simulink model "EPD629_WilliamsJ_AS06_Simulink"  (R2021b)
settings: Solver=VariableStepAuto  StartTime=0.0  StopTime=10.0  MaxStep=0.01  RelTol=1e-3
values from neighbouring files (symbols this model uses):
  AirGasConstant_kJpkgK = 0.287    [EPD629_WilliamsJ_AS06.m]
  AirToFuelEquivalenceRatio_frac = 1    [EPD629_WilliamsJ_AS06.m]
  AmbientPressure_kPa = 98    [EPD629_WilliamsJ_AS06.m]
  CrankAngleIVCToTDC_deg = 170    [EPD629_WilliamsJ_AS06.m]
  DischargeCoefficient_frac = 0.7    [EPD629_WilliamsJ_AS06.m]
  EngineDisplacement_L = 2.77    [EPD629_WilliamsJ_AS06.m]
  EngineInertia_kgm2 = 0.2    [EPD629_WilliamsJ_AS06.m]
  EngineMotoringFrictionData_Nm = Beta_0 + Beta_2*Omega_e.^2    [EPD629_WilliamsJ_AS06.m]
  EngineSpeedBreakpoints_rpm = 400:200:5000    [EPD629_WilliamsJ_AS06.m]
  FuelLowerHeatingValue_kJpkg = 44000    [EPD629_WilliamsJ_AS06.m]
  InletAirTemperature_K = 298    [EPD629_WilliamsJ_AS06.m]
  IntakeManifoldVolume_L = 5.8    [EPD629_WilliamsJ_AS06.m]
  ManifoldAirTemperature_K = 340    [EPD629_WilliamsJ_AS06.m]
  ManifoldPressureBreakpoints_kPa = 5:5:100    [EPD629_WilliamsJ_AS06.m]
  StoichiometricAFR_frac = 14.7    [EPD629_WilliamsJ_AS06.m]
  ThermodynamicEfficiencyData_frac = Eta_0 + Eta_1*Omega_e + Eta_2*Omega_e.^2    [EPD629_WilliamsJ_AS06.m]
  ThrottleAreaBreakpoints_pct = ThrottleAreaData_pct    [EPD629_WilliamsJ_AS06.m]
  ThrottleAreaData_pct = 100 * ThrottleArea_mm2 / WideOpenThrottleArea_mm2    [EPD629_WilliamsJ_AS06.m]
  ThrottleFlowFunctionData_frac = PR.^(1/RatioOfSpecificHeats_frac) .*      sqrt( 2 * RatioOfSpecificHeats_frac / (RatioOfSpecificHeats_frac - 1) .*      (1 - PR.^((RatioOfSpecificHeats_frac - 1) / RatioOfSpecificHeats_frac)) )    [EPD629_WilliamsJ_AS06.m]
  ThrottlePositionBreakpoints_pct = 0:100    [EPD629_WilliamsJ_AS06.m]
  ThrottlePositionData_pct = ThrottlePositionBreakpoints_pct    [EPD629_WilliamsJ_AS06.m]
  ThrottlePressureRatioBreakpoints_frac = 0:0.01:1    [EPD629_WilliamsJ_AS06.m]
  WideOpenThrottleArea_mm2 = ThrottleArea_mm2(end)    [EPD629_WilliamsJ_AS06.m]
undefined symbols (not defined in the file or in its folder): VolumetricEfficiencyData_frac
settings Model: Creator=Justin  LastModifiedBy=Justin

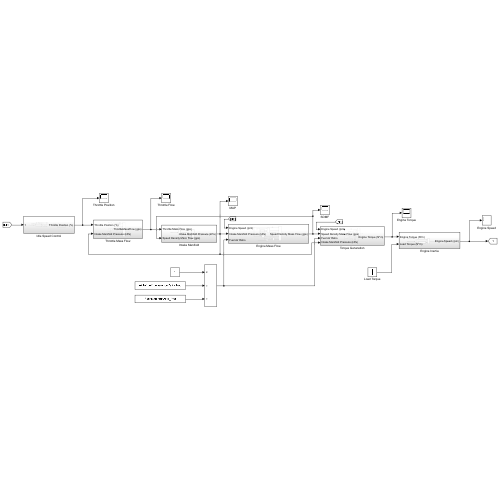
[thumbnail: Simulink's stored preview of the top-level diagram]
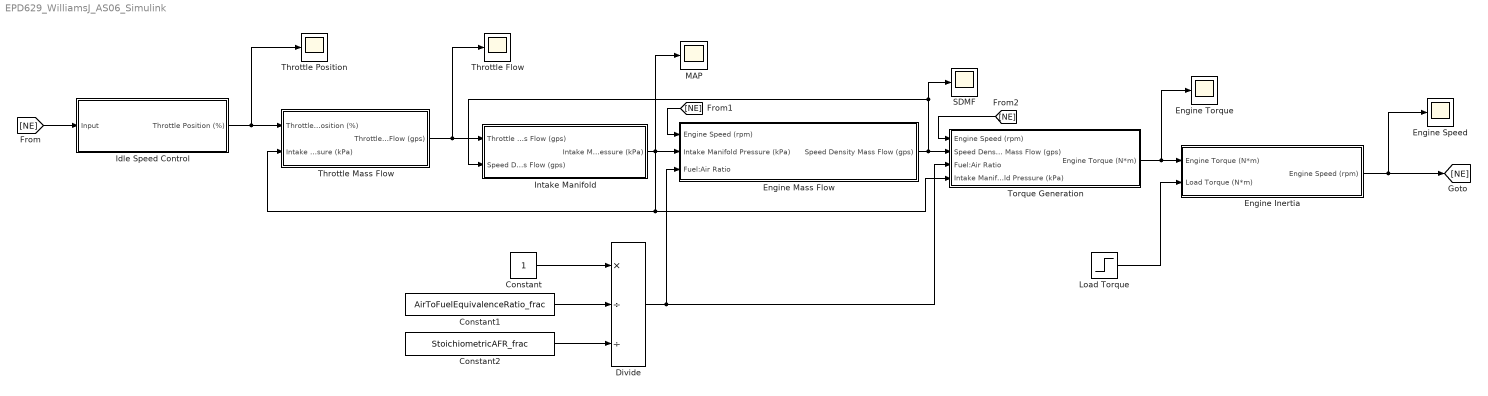
== system EPD629_WilliamsJ_AS06_Simulink ==
  Constant : Constant
  Constant1 : Constant  Value=AirToFuelEquivalenceRatio_frac
  Constant2 : Constant  Value=StoichiometricAFR_frac
  Divide : Product  Inputs=*//
  Engine Inertia : Subsystem
  Engine Mass Flow : Subsystem
  Engine Speed : Scope
  Engine Torque : Scope
  Idle Speed Control : Subsystem
  Intake Manifold : Subsystem
  Load Torque : Step  Time=5  Before=15  After=25  SampleTime=0
  MAP : Scope
  SDMF : Scope
  Throttle Flow : Scope
  Throttle Mass Flow : Subsystem
  Throttle Position : Scope
  Torque Generation : Subsystem
  wires:
  Constant/1 -> Divide/1
  Constant1/1 -> Divide/2
  Constant2/1 -> Divide/3
  Divide/1 -> Engine Mass Flow/3(Fuel:Air Ratio), Torque Generation/3(Fuel:Air Ratio)
  Load Torque/1 -> Engine Inertia/2(Load Torque (N*m))
  Idle Speed Control/1(Throttle Position (%)) -> Throttle Position/1, Throttle Mass Flow/1(Throttle Position (%))
  Throttle Mass Flow/1(ThrottleMassFlow (gps)) -> Throttle Flow/1, Intake Manifold/1(Throttle Mass Flow (gps))
  Intake Manifold/1(Intake Manifold Pressure (kPa)) -> Torque Generation/4(Intake Manifold Pressure (kPa)), Throttle Mass Flow/2(Intake Manifold Pressure (kPa)), MAP/1, Engine Mass Flow/2(Intake Manifold Pressure (kPa))
  Engine Mass Flow/1(Speed Density Mass Flow (gps)) -> SDMF/1, Intake Manifold/2(Speed Density Mass Flow (gps)), Torque Generation/2(Speed Density Mass Flow (gps))
  Torque Generation/1(Engine Torque (N*m)) -> Engine Torque/1, Engine Inertia/1(Engine Torque (N*m))
  Engine Inertia/1(Engine Speed (rpm)) -> [NE], Engine Speed/1
  [NE] -> Idle Speed Control/1(Input)
  [NE] -> Engine Mass Flow/1(Engine Speed (rpm))
  [NE] -> Torque Generation/1(Engine Speed (rpm))

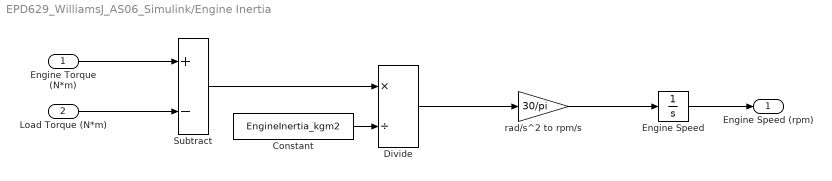
== system EPD629_WilliamsJ_AS06_Simulink/Engine Inertia ==
  Engine Torque (N*m) : Inport
  Load Torque (N*m) : Inport  Port=2
  Constant : Constant  Value=EngineInertia_kgm2
  Divide : Product  Inputs=*/
  Engine Speed : Integrator  InitialCondition=600  LimitOutput=on  UpperSaturationLimit=5000  LowerSaturationLimit=0
  Subtract : Sum  Inputs=+-
  rad/s^2 to rpm/s : Gain  Gain=30/pi
  Engine Speed (rpm) : Outport
  wires:
  Engine Torque (N*m)/1 -> Subtract/1
  Load Torque (N*m)/1 -> Subtract/2
  Subtract/1 -> Divide/1
  Constant/1 -> Divide/2
  Divide/1 -> rad/s^2 to rpm/s/1
  rad/s^2 to rpm/s/1 -> Engine Speed/1
  Engine Speed/1 -> Engine Speed (rpm)/1

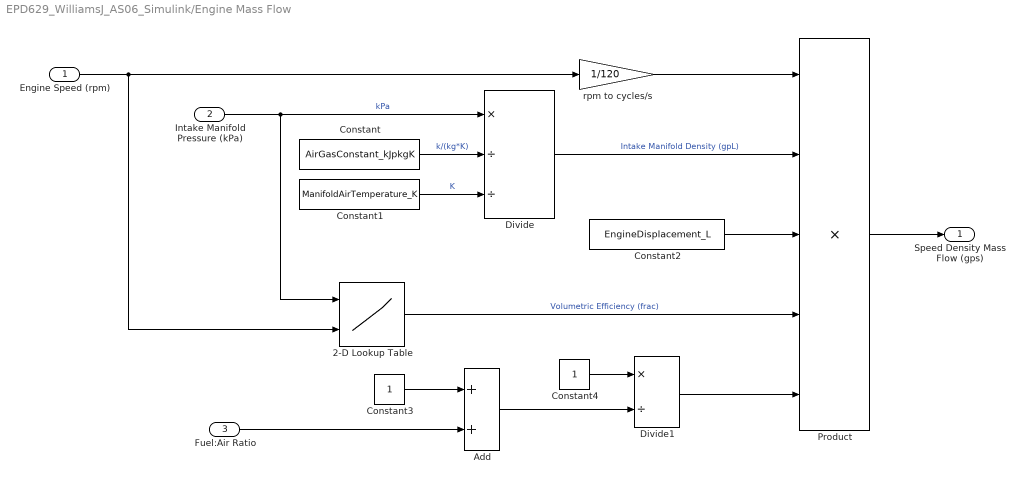
== system EPD629_WilliamsJ_AS06_Simulink/Engine Mass Flow ==
  Engine Speed (rpm) : Inport
  Intake Manifold Pressure (kPa) : Inport  Port=2
  Fuel:Air Ratio : Inport  Port=3
  2-D Lookup Table : Lookup_n-D  BreakpointsForDimension1=ManifoldPressureBreakpoints_kPa  BreakpointsForDimension2=EngineSpeedBreakpoints_rpm  Table=VolumetricEfficiencyData_frac  ExtrapMethod=Clip  UseLastTableValue=on  InternalRulePriority=Speed  RndMeth=Simplest  InputSameDT=on
      settings: InputPortMap=u0,u1
  Add : Sum
  Constant : Constant  Value=AirGasConstant_kJpkgK
  Constant1 : Constant  Value=ManifoldAirTemperature_K
  Constant2 : Constant  Value=EngineDisplacement_L
  Constant3 : Constant
  Constant4 : Constant
  Divide : Product  Inputs=*//
  Divide1 : Product  Inputs=*/
  Product : Product  Inputs=5
  rpm to cycles/s : Gain  Gain=1/120
  Speed Density Mass Flow (gps) : Outport
  wires:
  Engine Speed (rpm)/1 -> rpm to cycles/s/1, 2-D Lookup Table/2
  Intake Manifold Pressure (kPa)/1 -> Divide/1, 2-D Lookup Table/1  "kPa"
  Constant/1 -> Divide/2  "k/(kg*K)"
  Constant1/1 -> Divide/3  "K"
  rpm to cycles/s/1 -> Product/1
  Divide/1 -> Product/2  "Intake Manifold Density (gpL)"
  Constant2/1 -> Product/3
  2-D Lookup Table/1 -> Product/4  "Volumetric Efficiency (frac)"
  Constant3/1 -> Add/1
  Fuel:Air Ratio/1 -> Add/2
  Constant4/1 -> Divide1/1
  Add/1 -> Divide1/2
  Divide1/1 -> Product/5
  Product/1 -> Speed Density Mass Flow (gps)/1

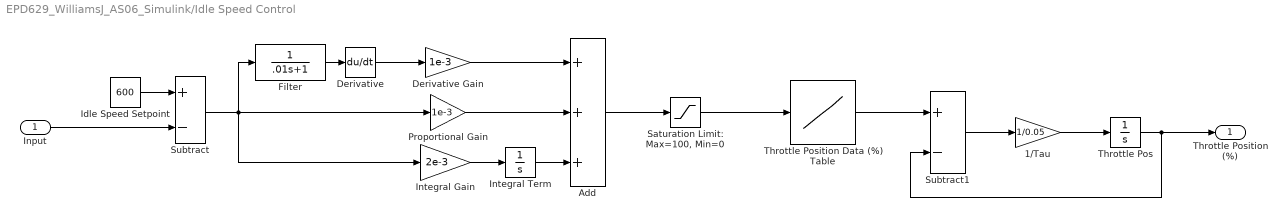
== system EPD629_WilliamsJ_AS06_Simulink/Idle Speed Control ==
  Input : Inport
  1/Tau : Gain  Gain=1/0.05
  Add : Sum  Inputs=+++
  Derivative : Derivative
  Derivative Gain : Gain  Gain=1e-3
  Filter : TransferFcn  Denominator=[.01 1]
  Idle Speed Setpoint : Constant  Value=600
  Integral Gain : Gain  Gain=2e-3
  Integral Term : Integrator  InitialCondition=0.6  LimitOutput=on  UpperSaturationLimit=100  LowerSaturationLimit=0
  Proportional Gain : Gain  Gain=1e-3
  "Saturation Limit: Max=100, Min=0" : Saturate  UpperLimit=100  LowerLimit=0
  Subtract : Sum  Inputs=+-
  Subtract1 : Sum  Inputs=+-
  Throttle Pos : Integrator  InitialCondition=1.7  LimitOutput=on  UpperSaturationLimit=100  LowerSaturationLimit=0
  Throttle Position Data (%) Table : Lookup_n-D  NumberOfTableDimensions=1  BreakpointsForDimension1=ThrottleAreaBreakpoints_pct  Table=ThrottlePositionData_pct  ExtrapMethod=Clip  UseLastTableValue=on  InternalRulePriority=Speed  RndMeth=Simplest  InputSameDT=on
  Throttle Position (%) : Outport
  wires:
  Idle Speed Setpoint/1 -> Subtract/1
  Filter/1 -> Derivative/1
  Subtract/1 -> Integral Gain/1, Filter/1, Proportional Gain/1
  Derivative/1 -> Derivative Gain/1
  Derivative Gain/1 -> Add/1
  Proportional Gain/1 -> Add/2
  Integral Gain/1 -> Integral Term/1
  Integral Term/1 -> Add/3
  Input/1 -> Subtract/2
  Add/1 -> "Saturation Limit: Max=100, Min=0"/1
  "Saturation Limit: Max=100, Min=0"/1 -> Throttle Position Data (%) Table/1
  Throttle Position Data (%) Table/1 -> Subtract1/1
  Subtract1/1 -> 1/Tau/1
  1/Tau/1 -> Throttle Pos/1
  Throttle Pos/1 -> Subtract1/2, Throttle Position (%)/1

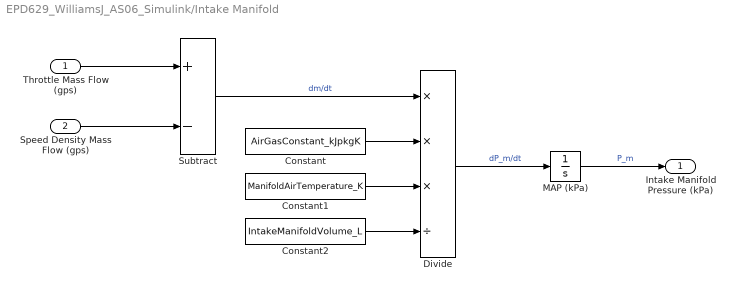
== system EPD629_WilliamsJ_AS06_Simulink/Intake Manifold ==
  Throttle Mass Flow (gps) : Inport
  Speed Density Mass Flow (gps) : Inport  Port=2
  Constant : Constant  Value=AirGasConstant_kJpkgK
  Constant1 : Constant  Value=ManifoldAirTemperature_K
  Constant2 : Constant  Value=IntakeManifoldVolume_L
  Divide : Product  Inputs=***/
  MAP (kPa) : Integrator  InitialCondition=33.5  LimitOutput=on  UpperSaturationLimit=110  LowerSaturationLimit=10
  Subtract : Sum  Inputs=+-
  Intake Manifold Pressure (kPa) : Outport
  wires:
  Throttle Mass Flow (gps)/1 -> Subtract/1
  Speed Density Mass Flow (gps)/1 -> Subtract/2
  Subtract/1 -> Divide/1  "dm/dt"
  Constant/1 -> Divide/2
  Constant1/1 -> Divide/3
  Constant2/1 -> Divide/4
  Divide/1 -> MAP (kPa)/1  "dP_m/dt"
  MAP (kPa)/1 -> Intake Manifold Pressure (kPa)/1  "P_m"

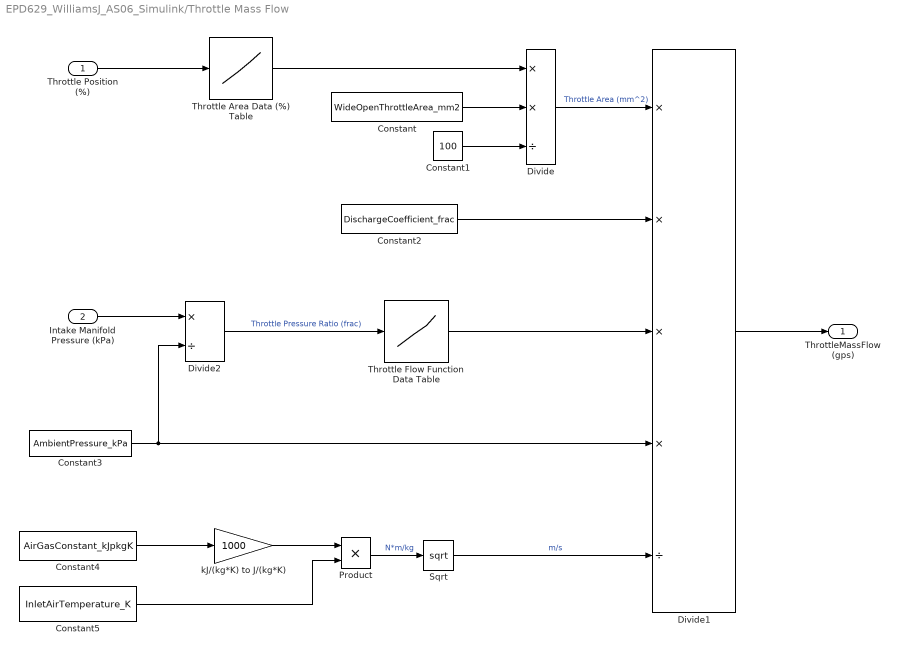
== system EPD629_WilliamsJ_AS06_Simulink/Throttle Mass Flow ==
  Throttle Position (%) : Inport
  Intake Manifold Pressure (kPa) : Inport  Port=2
  Constant : Constant  Value=WideOpenThrottleArea_mm2
  Constant1 : Constant  Value=100
  Constant2 : Constant  Value=DischargeCoefficient_frac
  Constant3 : Constant  Value=AmbientPressure_kPa
  Constant4 : Constant  Value=AirGasConstant_kJpkgK
  Constant5 : Constant  Value=InletAirTemperature_K
  Divide : Product  Inputs=**/
  Divide1 : Product  Inputs=****/
  Divide2 : Product  Inputs=*/
  Product : Product
  Sqrt : Sqrt  SaturateOnIntegerOverflow=on
  Throttle Area Data (%) Table : Lookup_n-D  NumberOfTableDimensions=1  BreakpointsForDimension1=ThrottlePositionBreakpoints_pct  Table=ThrottleAreaData_pct  ExtrapMethod=Clip  UseLastTableValue=on  InternalRulePriority=Speed  RndMeth=Simplest  InputSameDT=on
  Throttle Flow Function Data Table : Lookup_n-D  NumberOfTableDimensions=1  BreakpointsForDimension1=ThrottlePressureRatioBreakpoints_frac  Table=ThrottleFlowFunctionData_frac  ExtrapMethod=Clip  UseLastTableValue=on  InternalRulePriority=Speed  RndMeth=Simplest  InputSameDT=on
  kJ/(kg*K) to J/(kg*K) : Gain  Gain=1000
  ThrottleMassFlow (gps) : Outport
  wires:
  Throttle Position (%)/1 -> Throttle Area Data (%) Table/1
  Throttle Area Data (%) Table/1 -> Divide/1
  Constant/1 -> Divide/2
  Constant1/1 -> Divide/3
  Divide/1 -> Divide1/1  "Throttle Area (mm^2)"
  Constant2/1 -> Divide1/2
  Intake Manifold Pressure (kPa)/1 -> Divide2/1
  Constant3/1 -> Divide2/2, Divide1/4
  Throttle Flow Function Data Table/1 -> Divide1/3
  Divide2/1 -> Throttle Flow Function Data Table/1  "Throttle Pressure Ratio (frac)"
  Constant4/1 -> kJ/(kg*K) to J/(kg*K)/1
  kJ/(kg*K) to J/(kg*K)/1 -> Product/1
  Constant5/1 -> Product/2
  Product/1 -> Sqrt/1  "N*m/kg"
  Sqrt/1 -> Divide1/5  "m/s"
  Divide1/1 -> ThrottleMassFlow (gps)/1

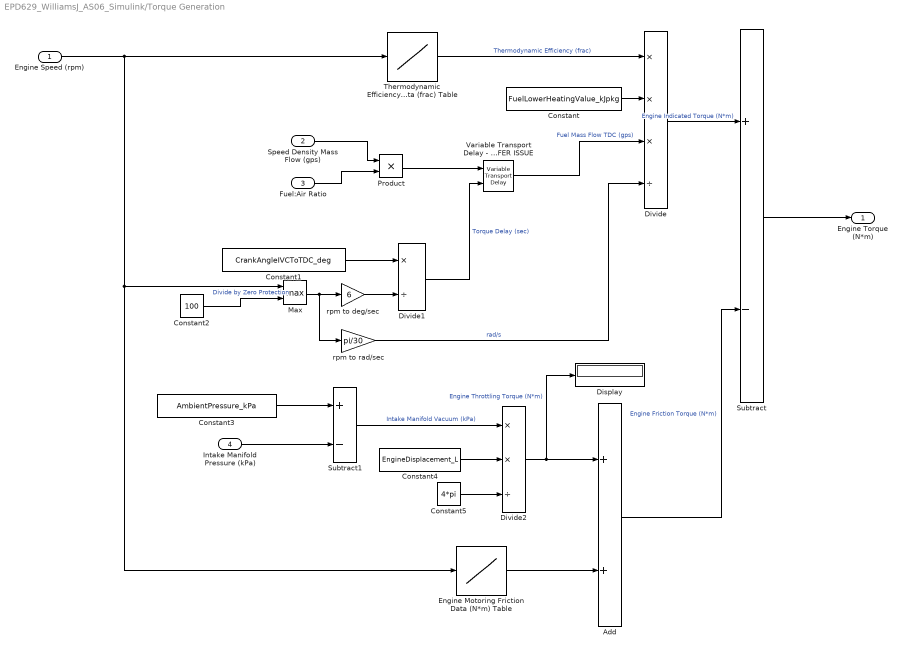
== system EPD629_WilliamsJ_AS06_Simulink/Torque Generation ==
  Engine Speed (rpm) : Inport
  Speed Density Mass Flow (gps) : Inport  Port=2
  Fuel:Air Ratio : Inport  Port=3
  Intake Manifold Pressure (kPa) : Inport  Port=4
  Add : Sum
  Constant : Constant  Value=FuelLowerHeatingValue_kJpkg
  Constant1 : Constant  Value=CrankAngleIVCToTDC_deg
  Constant2 : Constant  Value=100
  Constant3 : Constant  Value=AmbientPressure_kPa
  Constant4 : Constant  Value=EngineDisplacement_L
  Constant5 : Constant  Value=4*pi
  Display : Display
  Divide : Product  Inputs=***/
  Divide1 : Product  Inputs=*/
  Divide2 : Product  Inputs=**/
  Engine Motoring Friction Data (N*m) Table : Lookup_n-D  NumberOfTableDimensions=1  BreakpointsForDimension1=EngineSpeedBreakpoints_rpm  Table=EngineMotoringFrictionData_Nm  ExtrapMethod=Clip  UseLastTableValue=on  InternalRulePriority=Speed  RndMeth=Simplest  InputSameDT=on
  Max : MinMax  Function=max  Inputs=2
  Product : Product
  Subtract : Sum  Inputs=+-
  Subtract1 : Sum  Inputs=+-
  Thermodynamic Efficiency Data (frac) Table : Lookup_n-D  NumberOfTableDimensions=1  BreakpointsForDimension1=EngineSpeedBreakpoints_rpm  Table=ThermodynamicEfficiencyData_frac  ExtrapMethod=Clip  UseLastTableValue=on  InternalRulePriority=Speed  RndMeth=Simplest  InputSameDT=on
  "Variable Transport Delay - BUFFER ISSUE " : VariableTransportDelay  VariableDelayType=Variable transport delay  MaximumDelay=10  InitialOutput=0.166
  rpm to deg/sec : Gain  Gain=6
  rpm to rad/sec : Gain  Gain=pi/30
  Engine Torque (N*m) : Outport
  wires:
  Engine Speed (rpm)/1 -> Engine Motoring Friction Data (N*m) Table/1, Max/1, Thermodynamic Efficiency Data (frac) Table/1
  Thermodynamic Efficiency Data (frac) Table/1 -> Divide/1  "Thermodynamic Efficiency (frac)"
  Constant/1 -> Divide/2
  Speed Density Mass Flow (gps)/1 -> Product/1
  Fuel:Air Ratio/1 -> Product/2
  Product/1 -> "Variable Transport Delay - BUFFER ISSUE "/1
  "Variable Transport Delay - BUFFER ISSUE "/1 -> Divide/3  "Fuel Mass Flow TDC (gps)"
  Constant1/1 -> Divide1/1
  Constant2/1 -> Max/2  "Divide by Zero Protection"
  Max/1 -> rpm to rad/sec/1, rpm to deg/sec/1
  rpm to deg/sec/1 -> Divide1/2
  Divide1/1 -> "Variable Transport Delay - BUFFER ISSUE "/2  "Torque Delay (sec)"
  rpm to rad/sec/1 -> Divide/4  "rad/s"
  Divide/1 -> Subtract/1  "Engine Indicated Torque (N*m)"
  Constant3/1 -> Subtract1/1
  Intake Manifold Pressure (kPa)/1 -> Subtract1/2
  Subtract1/1 -> Divide2/1  "Intake Manifold Vacuum (kPa)"
  Constant4/1 -> Divide2/2
  Constant5/1 -> Divide2/3
  Engine Motoring Friction Data (N*m) Table/1 -> Add/2
  Divide2/1 -> Display/1, Add/1  "Engine Throttling Torque (N*m)"
  Add/1 -> Subtract/2  "Engine Friction Torque (N*m)"
  Subtract/1 -> Engine Torque (N*m)/1
